simulink model "twoTank"  (R2021a)
settings: Solver=FixedStepAuto  StartTime=0.0  StopTime=timeFinal  FixedStep=timeStepMax  MaxStep=timeStepMax  RelTol=1e-3
model workspace (MAT data in the model file):
  x0 = 5
  y0 = 5
undefined symbols (not defined in the file): a1, a2
settings Model: SimulationMode=accelerator  Creator=amit  LastModifiedBy=amit
settings DataIOCC: ExternalInput=ds  LoadExternalInput=on

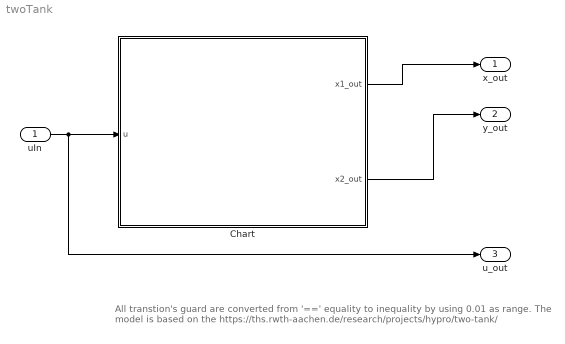
== system twoTank ==
  note: All transtion's guard are converted from '==' equality to inequality by using 0.01 as range.
      | The model is based on the https://ths.rwth-aachen.de/research/projects/hypro/two-tank/
  uIn : Inport
  Chart : Stateflow chart  TreatAsAtomicUnit=on
  x_out : Outport  SignalName=x1Out
  y_out : Outport  Port=2  SignalName=x2Out
  u_out : Outport  Port=3  SignalName=x3Out
  wires:
  Chart/1(x1_out) -> x_out/1
  Chart/2(x2_out) -> y_out/1
  uIn/1 -> u_out/1, Chart/1(u)

== stateflow chart twoTank/Chart ==
  settings: updateMethod=CONTINUOUS  executeAtInitialization=1
  state off_off
    du:  % derivatives
    x1_dot = -1.0 * x1 - 2 + u;
    x2_dot = 1.0 * x1 + u;
    exit:
    x1_out=x1;
    x2_out=x2;
  state on_off
    du:  % derivatives
    x1_dot = -1.0 * x1 + 3 + u;
    x2_dot = 1.0 * x1 + u;
    exit:
    x1_out=x1;
    x2_out=x2;
  state off_on
    du:  % derivatives
    x1_dot = -1.0 * x1 - 2 + u;
    x2_dot = 1.0 * x1 - 1.0 * x2 - 5 + u;
    exit:
    x1_out=x1;
    x2_out=x2;
  state on_on
    du:
    x1_dot =  -1.0 * x1 + 3 + u;
    x2_dot = 1.0 * x1 - 1.0 * x2 - 5 + u;
    exit:
    x1_out=x1;
    x2_out=x2;
  (default) -> off_off : {x1=a1; x2=a2;}
  on_off -> on_off [order 2] : [x2<=1]{x1=x1; x2=x2;}
  off_off -> off_off [order 3] : [x1>=-1 & x2<=1]{x1=x1; x2=x2;}
  off_off -> on_off [order 1] : [x1>= -1 - 0.01 & x1<= -1 + 0.01]{x1=x1; x2=x2;}
  on_off -> off_on [order 1] : [x2>=1]{x1=x1; x2=x2;}
  off_off -> off_on [order 2] : [x2>= 1 - 0.01 & x2<= 1 + 0.01]{x1=x1; x2=x2;}
  off_on -> off_off [order 2] : [x2>= 0 - 0.01 & x2<= 0 + 0.01]{x1=x1; x2=x2;}
  on_on -> on_off [order 1] : [x2>= 0- 0.01 & x2<= 0 + 0.01]{x1=x1; x2=x2;}
  off_on -> off_on [order 3] : [x1>=-1 & x2>=0]{x1=x1; x2=x2;}
  on_on -> off_on [order 2] : [x1>=1-0.01 & x1<=1 +0.01]{x1=x1; x2=x2;}
  off_on -> on_on [order 1] : [x1>= -1 - 0.01 & x1<= -1 + 0.01]{x1=x1; x2=x2;}
  on_on -> on_on [order 3] : [x1<=1 & x2>=0]{x1=x1; x2=x2;}
  data: a1 parameter; x1_out output; x2_out output; x1 local; x2 local; u input; a2 parameter
  data x1 settings: updateMethod=SF_CONTINUOUS_TIME_DATA
  data x2 settings: updateMethod=SF_CONTINUOUS_TIME_DATA
